simulink model "KF_to_play_with"  (R2020a)
settings: Solver=ode1  StartTime=0.0  StopTime=10.0  FixedStep=0.001  MaxStep=.001  RelTol=1e-3  EnableMultiTasking=on
values from neighbouring files (symbols this model uses):
  A = [0 1 0 ... (first row only)    [KF3_Script.m]    (also in KF_Script.m = [0 1; LQG_Script.m)
  B = [0 Kt/J 0]'    [KF3_Script.m]    (also in KF_Script.m = [0 Kt/J]'; LQG_Script.m)
  C = [1 0 0]    [KF3_Script.m]    (also in KF_Script.m = [1 0]; LQG_Script.m)
  D = 0    [KF3_Script.m]    (also in KF_Script.m; LQG_Script.m)
  Fes = F-L*H    [KF3_Script.m]    (also in KF_Script.m; LQG_Script.m)
  L = (dlqr(F',H',Q,R))'    [KF3_Script.m]    (also in KF_Script.m; LQG_Script.m)
undefined symbols (not defined in the file or in its folder): G
settings Model: Creator=oboe  LastModifiedBy=Saverio
settings DataIOCC: LimitDataPoints=on  SaveFormat=Array  ReturnWorkspaceOutputs=off
settings OptimizationCC: LifeSpan=inf
settings DebuggingCC: SolverPrmCheckMsg=warning  SFUnexpectedBacktrackingDiag=warning  SFNoUnconditionalDefaultTransitionDiag=warning  SFExecutionAtInitializationDiag=none  ArithmeticOperatorsInVariantConditions=warning
settings HardwareCC: ProdBitPerPointer=32  ProdBitPerSizeT=32  ProdBitPerPtrDiffT=32  ProdLargestAtomicFloat=None  ProdIntDivRoundTo=Undefined  ProdEndianess=Unspecified  ProdWordSize=32  ProdHWDeviceType=32-bit Generic
settings ModelReferenceCC: PropagateSignalLabelsOutOfModel=off
settings SFSimCC: SimUseLocalCustomCode=off  CustomCodeUndefinedFunction=UseInterfaceOnly
settings RTWCC: RTWUseLocalCustomCode=off
settings CodeAppCC: StateflowObjectComments=on
settings GRTTargetCC: TargetLangStandard=C89/C90 (ANSI)
settings ConfigComp: CovMetricSettings=dw  CovHtmlReporting=on  CovSaveCumulativeToWorkspaceVar=on  CovSaveSingleToWorkspaceVar=on  CovExternalEMLEnable=off  CovSFcnEnable=off

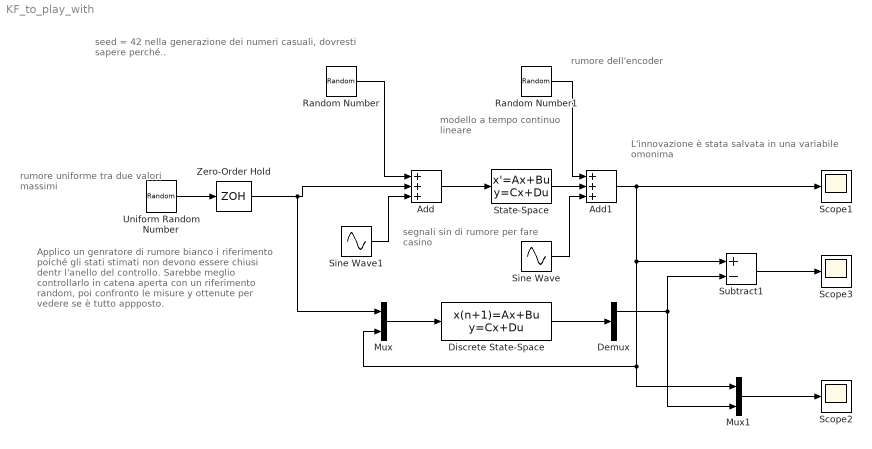
== system KF_to_play_with ==
  note: seed = 42 nella generazione dei numeri casuali,
      | dovresti sapere perché..
  note: rumore uniforme tra
      | due valori massimi
  note: Applico un genratore di rumore bianco i riferimento
      | poiché gli stati stimati non devono essere chiusi dentr
      | l'anello del controllo. Sarebbe meglio controllarlo in catena
      | aperta con un riferimento random, poi confronto le misure y
      | ottenute per vedere se è tutto appposto.
  note: modello a tempo continuo
      | lineare
  note: rumore dell'encoder
  note: L'innovazione è stata  salvata in una
      | variabile omonima
  note: segnali sin di rumore
      | per fare casino
  Add : Sum  Inputs=+++
  Add1 : Sum  Inputs=+++
  Demux : Demux  Outputs=2
  Discrete State-Space : DiscreteStateSpace  A=Fes  B=[G L]  C=eye(2)  D=zeros(2,2)  SampleTime=.001
  Mux : Mux  Inputs=2
  Mux1 : Mux  Inputs=2
  Random Number : RandomNumber  Variance=(10/2^12)^2/12  Seed=42  SampleTime=0.001
  Random Number1 : RandomNumber  Variance=(2*pi/2000)^2/12  Seed=42*42  SampleTime=0.001
  Scope1 : Scope
  Scope2 : Scope
  Scope3 : Scope
  Sine Wave : Sin  Amplitude=0  Frequency=500  SampleTime=0
  Sine Wave1 : Sin  Amplitude=2  Frequency=1000  SampleTime=0
  State-Space : StateSpace  A=A  B=B  C=C  D=D  InitialCondition=0
  Subtract1 : Sum  Inputs=+-
  Uniform Random Number : UniformRandomNumber  Minimum=-.1  Maximum=.1  Seed=42  SampleTime=0.001
  Zero-Order Hold : ZeroOrderHold  SampleTime=0.001
  wires:
  Uniform Random Number/1 -> Zero-Order Hold/1
  Mux/1 -> Discrete State-Space/1
  Discrete State-Space/1 -> Demux/1
  Demux/1 -> Mux1/2, Subtract1/2
  Mux1/1 -> Scope2/1
  Subtract1/1 -> Scope3/1
  Random Number1/1 -> Add1/1
  Add1/1 -> Mux/2, Mux1/1, Subtract1/1, Scope1/1
  Zero-Order Hold/1 -> Mux/1, Add/2
  Random Number/1 -> Add/1
  State-Space/1 -> Add1/2
  Sine Wave/1 -> Add1/3
  Add/1 -> State-Space/1
  Sine Wave1/1 -> Add/3
